simulink model "n_liniarisiert"  (R2015a)
settings: Solver=ode45  StartTime=0.0  StopTime=25.0  RelTol=1e-3
settings Model: Creator=lustoppe  LastModifiedBy=lustoppe

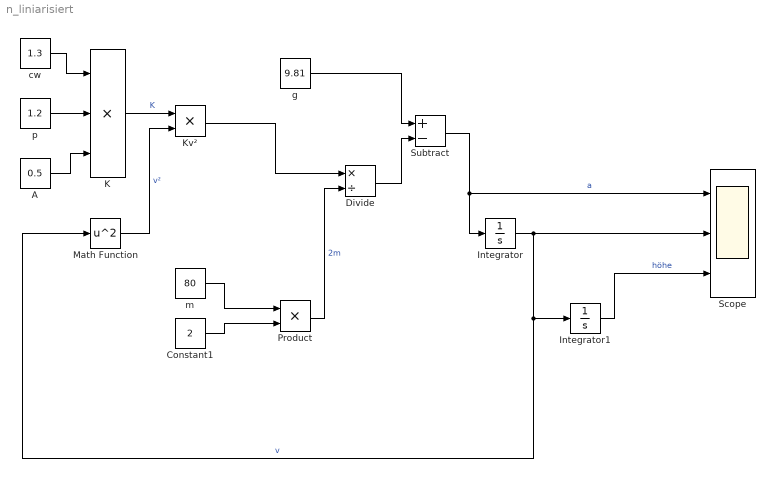
== system n_liniarisiert ==
  "A " : Constant  Value=0.5
  Constant1 : Constant  Value=2
  Divide : Product  Inputs=*/
  Integrator : Integrator
  Integrator1 : Integrator
  K : Product  Inputs=3
  Kv² : Product
  Math Function : Math  Operator=square  SaturateOnIntegerOverflow=on
  Product : Product
  Scope : Scope  NumInputPorts=3
      settings: YMin=-5~-5~-5  YMax=5~5~5
  Subtract : Sum  Inputs=+-
  "cw " : Constant  Value=1.3
  g : Constant  Value=9.81
  "m " : Constant  Value=80
  "p " : Constant  Value=1.2
  wires:
  "cw "/1 -> K/1
  "p "/1 -> K/2
  "A "/1 -> K/3
  Subtract/1 -> Scope/1, Integrator/1  "a"
  g/1 -> Subtract/1
  Product/1 -> Divide/2  "2m"
  "m "/1 -> Product/1
  Constant1/1 -> Product/2
  Divide/1 -> Subtract/2
  Integrator1/1 -> Scope/3  "höhe"
  Integrator/1 -> Math Function/1, Integrator1/1, Scope/2  "v"
  K/1 -> Kv²/1  "K"
  Math Function/1 -> Kv²/2  "v²"
  Kv²/1 -> Divide/1
